simulink model "Experimento3"  (R2021a)
settings: Solver=VariableStepAuto  StartTime=0.0  StopTime=1/60  RelTol=1e-3
libraries: spsRMSLib x8, spsVoltageMeasurementLib x4, spsACVoltageSourceLib x2, spsGroundLib x2, spsDCVoltageSourceLib x1, spsSeriesRLCBranchLib x1, spspowerguiLib x1
settings Model: Creator=55329  LastModifiedBy=55329

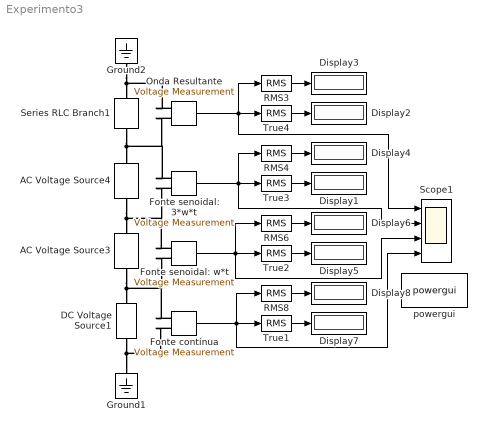
== system Experimento3 ==
  AC Voltage Source3 : spsACVoltageSourceLib/AC Voltage Source  Amplitude=169.71  Phase=0  Frequency=(2*pi*60)  SampleTime=0  Measurements=None  BusType=swing  Pref=10e3  Qref=0  Qmin=-inf  Qmax=+inf
  AC Voltage Source4 : spsACVoltageSourceLib/AC Voltage Source  Amplitude=84.85  Phase=0  Frequency=3*(2*pi*60)  SampleTime=0  Measurements=None  BusType=swing  Pref=10e3  Qref=0  Qmin=-inf  Qmax=+inf
  DC Voltage Source1 : spsDCVoltageSourceLib/DC Voltage Source  Amplitude=30  Measurements=None
  Display{1..8} (8 alike) : Display
  Fonte contínua : spsVoltageMeasurementLib/Voltage Measurement  PhasorSimulation=off  OutputType=Complex  PSBequivalent=0
  Fonte senoidal: 3*w*t : spsVoltageMeasurementLib/Voltage Measurement  PhasorSimulation=off  OutputType=Complex  PSBequivalent=0
  Fonte senoidal: w*t : spsVoltageMeasurementLib/Voltage Measurement  PhasorSimulation=off  OutputType=Complex  PSBequivalent=0
  Ground1 : spsGroundLib/Ground  LConnTagsString=a
  Ground2 : spsGroundLib/Ground  LConnTagsString=a
  Onda Resultante : spsVoltageMeasurementLib/Voltage Measurement  PhasorSimulation=off  OutputType=Complex  PSBequivalent=0
  RMS{3..4,6,8} (4 alike) : spsRMSLib/RMS  TrueRMS=off  Freq=60  RMSInit=0  Ts=0
  Scope1 : Scope  NumInputPorts=4
  Series RLC Branch1 : spsSeriesRLCBranchLib/Series RLC Branch  LConnTagsString=__new0  RConnTagsString=__new0  BranchType=R  Resistance=1  Inductance=0  SetiL0=off  InitialCurrent=0  Capacitance=0  Setx0=off  InitialVoltage=0  Measurements=None
  True{1..4} (4 alike) : spsRMSLib/RMS  TrueRMS=on  Freq=60  RMSInit=0  Ts=0
  powergui : spspowerguiLib/powergui  Priority=1  SimulationMode=Discrete  SampleTime=1/60/1000  frequency=60  Iterations=50  frequencyindice=0  Pbase=100e6  ErrMax=1e-4  UnitsV=kV  UnitsW=MW  buscounter=0  FunctionMessages=off  echomessages=off  EnableUseOfTLC=off  CurrentSourceSwitches=off  DisableSnubberDevices=off  DisableRonSwitches=off  DisableVfSwitches=off  DisplayEquations=off  AutomaticDiscreteSolvers=off  SolverType=Tustin  Interpol=off  ExternalGateDelay=off  methode=off  Ts=0  x0status=blocks  SPID=off  SwTol=0  HookPort=off  NonlinearTolerance=1e-4  nMaxIteration=100  ContinueOnMaxIteration=off  RestoreLinks=warning  ResistiveCurrentMeasurement=off  Frange=[0:2:500]  Ylog=off  Xlog=on  ShowGrid=off  save=off  variable=ZData  structure=simout  ZoomFFT=off  StartTime=0  cycles=10  DisplayStyle=2  fundamental=50  FreqAxis=on  MaxFrequency=2000  frequencyindicesteady=1  RmsSteady=1  display=off
  wires:
  True4/1 -> Display2/1
  RMS3/1 -> Display3/1
  Onda Resultante/1 -> RMS3/1, True4/1, Scope1/1
  Fonte senoidal: 3*w*t/1 -> RMS4/1, True3/1, Scope1/2
  Fonte senoidal: w*t/1 -> RMS6/1, True2/1, Scope1/3
  Fonte contínua/1 -> Scope1/4, True1/1, RMS8/1
  True3/1 -> Display1/1
  RMS4/1 -> Display4/1
  True2/1 -> Display5/1
  RMS6/1 -> Display6/1
  True1/1 -> Display7/1
  RMS8/1 -> Display8/1
  connections:
  AC Voltage Source4/LConn1 -- Fonte senoidal: w*t/LConn1 -- Fonte senoidal: 3*w*t/LConn2 -- AC Voltage Source3/RConn1
  DC Voltage Source1/LConn1 -- Fonte contínua/LConn2 -- Ground1/LConn1
  AC Voltage Source3/LConn1 -- Fonte senoidal: w*t/LConn2 -- Fonte contínua/LConn1 -- DC Voltage Source1/RConn1
  Series RLC Branch1/RConn1 -- Onda Resultante/LConn2 -- Fonte senoidal: 3*w*t/LConn1 -- AC Voltage Source4/RConn1
  Ground2/LConn1 -- Onda Resultante/LConn1 -- Series RLC Branch1/LConn1
